simulink model "simulink_problem_3_5_148"  (R2017b)
settings: Solver=VariableStepAuto  StartTime=0.0  StopTime=10.0  RelTol=1e-3
settings Model: Creator=ghost  LastModifiedBy=ghost

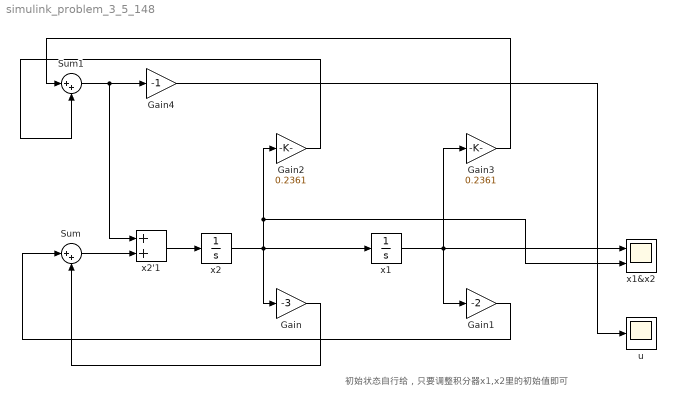
== system simulink_problem_3_5_148 ==
  note: 初始状态自行给，只要调整积分器x1,x2里的初始值即可
  Gain : Gain  Gain=-3
  Gain1 : Gain  Gain=-2
  Gain2 : Gain  Gain=0.2361
  Gain3 : Gain  Gain=0.2361
  Gain4 : Gain  Gain=-1
  Sum : Sum  Inputs=|++
  Sum1 : Sum  Inputs=|++
  u : Scope
  "x1 " : Integrator  InitialCondition=5
  x1&x2 : Scope  NumInputPorts=2
  "x2 " : Integrator  InitialCondition=5
  x2'1 : Sum
  wires:
  "x2 "/1 -> "x1 "/1, x1&x2/2, Gain2/1, Gain/1
  Gain/1 -> Sum/2
  "x1 "/1 -> Gain3/1, x1&x2/1, Gain1/1
  Gain1/1 -> Sum/1
  x2'1/1 -> "x2 "/1
  Sum/1 -> x2'1/2
  Gain2/1 -> Sum1/2
  Gain3/1 -> Sum1/1
  Sum1/1 -> Gain4/1, x2'1/1
  Gain4/1 -> u/1
